simulink model "Testt"  (R2012b)
settings: Solver=ode45  StartTime=0.0  StopTime=SimTime  RelTol=1e-3
undefined symbols (not defined in the file or in its folder): SimTime, Theta0, Theta1
settings Model: Creator=Alma  LastModifiedBy=Alma

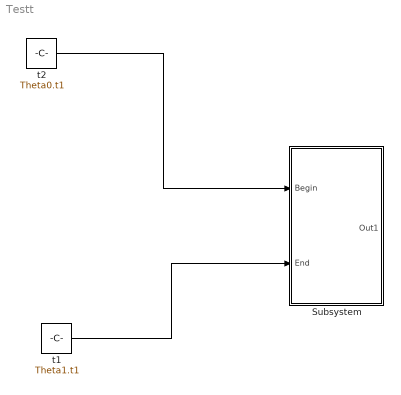
== system Testt ==
  Subsystem : Subsystem
  t1 : Constant  Value=Theta1.t1
  t2 : Constant  Value=Theta0.t1
  wires:
  t2/1 -> Subsystem/1(Begin)
  t1/1 -> Subsystem/2("End ")

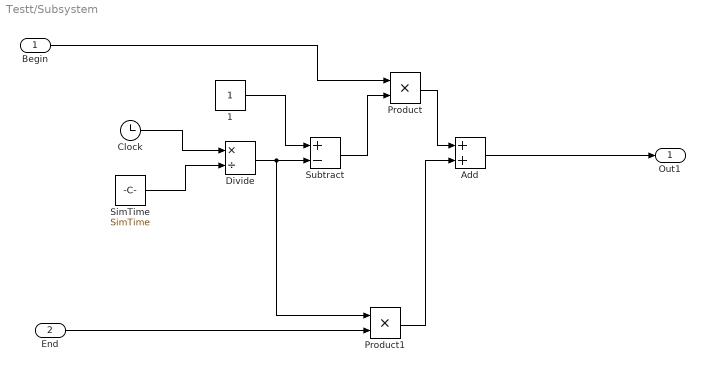
== system Testt/Subsystem ==
  Begin : Inport
  "End " : Inport  Port=2
  1 : Constant
  Add : Sum
  Clock : Clock
  Divide : Product  Inputs=*/
  Product : Product  RndMeth=Zero
  Product1 : Product  RndMeth=Zero
  "SimTime " : Constant  Value=SimTime
  Subtract : Sum  Inputs=+-
  Out1 : Outport
  wires:
  Product/1 -> Add/1
  Begin/1 -> Product/1
  Divide/1 -> Product1/1, Subtract/2
  1/1 -> Subtract/1
  Add/1 -> Out1/1
  "End "/1 -> Product1/2
  Subtract/1 -> Product/2
  Product1/1 -> Add/2
  Clock/1 -> Divide/1
  "SimTime "/1 -> Divide/2
